simulink model "physikalischeModelierung"  (R2014b)
settings: Solver=ode45  StartTime=0.0  StopTime=50  RelTol=1e-3
libraries: vrlib x2, cstblocks x1
settings Model: Creator=hollowman  LastModifiedBy=sigurd

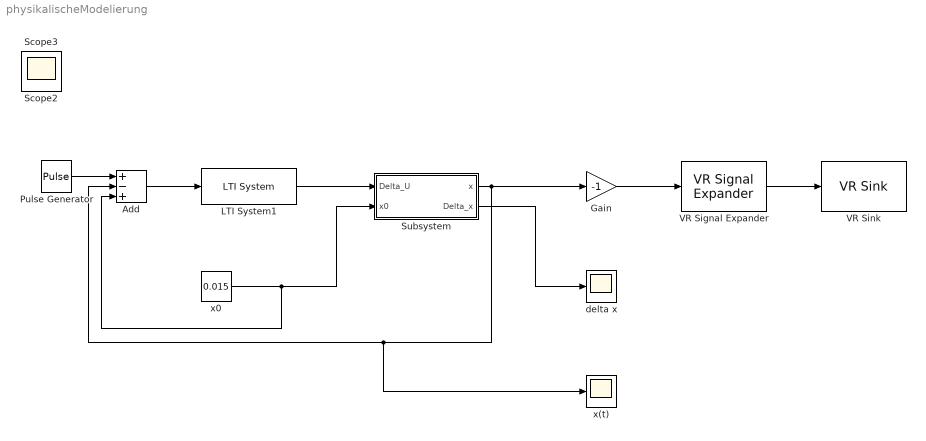
== system physikalischeModelierung ==
  Add : Sum  Inputs=+-+
  Gain : Gain  Gain=-1
  LTI System1 : cstblocks/LTI System  sys=C  IC=[]
  Pulse Generator : DiscretePulseGenerator  PulseType=Time based  Amplitude=0.001  Period=10  PulseWidth=50
  Subsystem : Subsystem
  VR Signal Expander : vrlib/VR Signal Expander  outwidth=3  outidx=[2]
  VR Sink : vrlib/VR Sink  InstantiateOnLoad=on  SampleTime=0.1  ViewEnable=on  RemoteChange=off  RemoteView=off  FieldsWritten=Kugel.translation.3.1.1.double  WorldFileName=Schwebekugel.WRL  AutoView=off  VideoDimensions=[]  AllowVariableSize=off  FigureProperties="{'Position', 'Name', 'Viewpoint', 'CameraBound', 'CameraDirection', 'CameraPosition', 'CameraUpVector', 'ZoomFactor', 'Antialiasing', 'Headlight', 'Lighting', 'NavPanel', 'Sound', 'StatusBar', 'Stereo3D', 'Stereo3DCameraOffset', 'Stereo3DHIT', 'ToolBar', 'Textures', 'Transparency', 'Triad', 'Wireframe', 'NavZones', 'NavMode', 'NavSpeed', 'CaptureFileFormat', 'CaptureFileName', 'Record2DCompressMethod', 'Record2DCompressQuality', 'Record2D', 'Record2DFileName', 'Record2DFPS'; [-1.6600000000000000e+02  -7.1700000000000000e+02   5.7600000000000000e+02   3.8000000000000000e+02], '', '_untitled_1', 'on', [0.0000000000000000e+00   0.0000000000000000e+00  -1.0000000000000000e+00], [0.0000000000000000e+00   0.0000000000000000e+00   0.0000000000000000e+00], [0.0000000000000000e+00   1.0000000000000000e+00   0.0000000000000000e+00], [1.0000000000000000e+00], 'on', 'on', 'on', 'halfbar', 'on', 'on', 'off', [1.0000000149011612e-01], [0.0000000000000000e+00], 'on', 'on', 'on', 'none', 'off', 'off', 'fly', 'normal', 'tif', '%f_anim_%n.tif', 'auto', [7.5000000000000000e+01], 'off', '%f_anim_%n.avi', 'auto'}"
  delta x : Scope
  x(t) : Scope
  x0 : Constant  Value=0.015
  Scope2 : Scope
      settings: YMin=0.0135  YMax=0.0175  MaxDataPoints=7500
  Scope3 : Scope
      settings: MaxDataPoints=7500
  wires:
  Pulse Generator/1 -> Add/1
  Add/1 -> LTI System1/1
  Gain/1 -> VR Signal Expander/1
  VR Signal Expander/1 -> VR Sink/1
  Subsystem/2(Delta_x) -> delta x/1
  LTI System1/1 -> Subsystem/1(Delta_U)
  x0/1 -> Add/3, Subsystem/2(x0)
  Subsystem/1(x) -> x(t)/1, Add/2, Gain/1

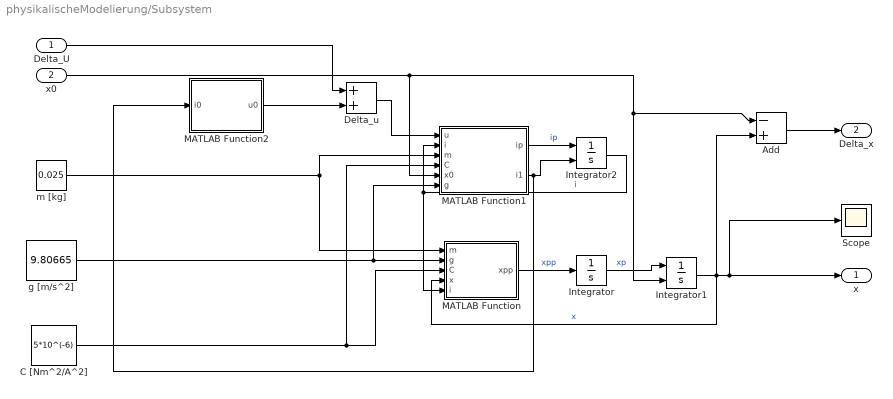
== system physikalischeModelierung/Subsystem ==
  Delta_U : Inport
  x0 : Inport  Port=2
  Add : Sum  Inputs=-+
  C [Nm^2/A^2] : Constant  Value=5*10^(-6)
  Delta_u : Sum
  Integrator : Integrator
  Integrator1 : Integrator  InitialConditionSource=external  InitialCondition=0.015
  Integrator2 : Integrator  InitialConditionSource=external  InitialCondition=3.3215
  MATLAB Function : MATLAB Function  TreatAsAtomicUnit=on
  MATLAB Function1 : MATLAB Function  TreatAsAtomicUnit=on
  MATLAB Function2 : MATLAB Function  TreatAsAtomicUnit=on
  Scope : Scope
      settings: SaveName=ScopeData2
  g [m/s^2] : Constant  Value=9.80665
  m [kg] : Constant  Value=0.025
  x : Outport
  Delta_x : Outport  Port=2
  wires:
  MATLAB Function/1(xpp) -> Integrator/1  "xpp"
  Integrator1/1 -> Add/2, Scope/1, x/1, MATLAB Function/4(x)  "x"
  Integrator/1 -> Integrator1/1  "xp"
  MATLAB Function1/1(ip) -> Integrator2/1  "ip"
  Integrator2/1 -> MATLAB Function/5(i), MATLAB Function1/2(i)  "i"
  Delta_U/1 -> Delta_u/1
  Delta_u/1 -> MATLAB Function1/1(u)
  MATLAB Function2/1(u0) -> Delta_u/2
  Add/1 -> Delta_x/1
  C [Nm^2/A^2]/1 -> MATLAB Function1/4(C), MATLAB Function/3(C)
  g [m/s^2]/1 -> MATLAB Function1/6(g), MATLAB Function/2(g)
  m [kg]/1 -> MATLAB Function1/3(m), MATLAB Function/1(m)
  x0/1 -> Integrator1/2, Add/1, MATLAB Function1/5(x0)
  MATLAB Function1/2(i1) -> MATLAB Function2/1(i0), Integrator2/2

== matlab function physikalischeModelierung/Subsystem/MATLAB Function1 ==
  data: u input; ip output; i input; i1 output; m input; C input; x0 input; g input
function [ip, i1] = fcn(u, i, m, C, x0, g)

R=3;
L=0.1;

ip = (u/L) - ((R*i)/L);
i1 = sqrt((m*g)/C) * x0;

== matlab function physikalischeModelierung/Subsystem/MATLAB Function ==
  data: m input; xpp output; g input; C input; x input; i input
function xpp = fcn(m, g, C, x, i)

xpp = g - ((C*i^2) / (x^2 * m));

== matlab function physikalischeModelierung/Subsystem/MATLAB Function2 ==
  data: u0 output; i0 input
function u0 = fcn(i0)
%#codegen
R=3;
u0 = R*i0;
